simulink model "moore_machine"  (R2020a)
settings: Solver=VariableStepAuto  StartTime=0.0  StopTime=20  RelTol=1e-3
settings Model: Creator=macharold  LastModifiedBy=Roland Varga
settings DataIOCC: FinalStateName=myOperPoint  InitialState=myOperPoint  LoadExternalInput=on  SaveFinalState=on  SaveOperatingPoint=on  ReturnWorkspaceOutputs=off
settings DebuggingCC: SignalResolutionControl=None  ArithmeticOperatorsInVariantConditions=warning
settings SFSimCC: SimUseLocalCustomCode=off  CustomCodeUndefinedFunction=UseInterfaceOnly
settings RTWCC: RTWUseLocalCustomCode=off

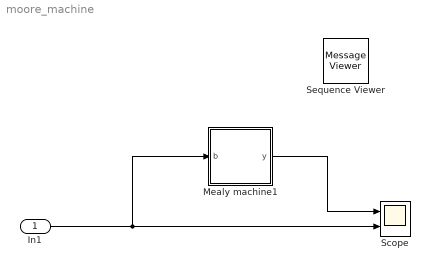
== system moore_machine ==
  In1 : Inport  SampleTime=1
  Mealy machine1 : Stateflow chart  TreatAsAtomicUnit=on
  Scope : Scope  NumInputPorts=2
  Sequence Viewer : MessageViewer  History=1000
  wires:
  In1/1 -> Mealy machine1/1(b), Scope/2
  Mealy machine1/1(y) -> Scope/1

== stateflow chart moore_machine/Mealy machine1 ==
  settings: sampleTime=1
  state S21
  state S20
  state S19
  state S1
  state S5
  state S6
  state S7
  state S8
  state S9
  state S10
  state S24
  state S25
  state S22
  state S14
  state S11
  state S13
  state S12
  state S26
  state S23
  state S15
  state S18
  state S17
  state S16
  state S28
  state S30
  state S31
  state S33
  state S34
  state S35
  state S36
  state S37
  state S38
  S16 -> S8 [order 1] : [b==1]{y=0}
  S21 -> S28 [order 2] : [b==0]{y=0}
  S19 -> S21 [order 2] : [b==1]
  S21 -> S13 [order 1] : [b==1]{y=0}
  S20 -> S28 [order 2] : [b==0]{y=0}
  S10 -> S19 [order 2] : [b==0]
  S19 -> S20 [order 1] : [b==0]
  S20 -> S18 [order 1] : [b==1]{y=0}
  S10 -> S10 [order 1] : [b==1]
  S1 -> S5 [order 2] : [b==1]
  S5 -> S6 [order 1] : [b==1]
  S6 -> S7 [order 1] : [b==1]{y=0}
  S7 -> S8 [order 1] : [b==1]
  S8 -> S9 [order 1] : [b==1]
  (default) -> S1 : {y=-1}
  S9 -> S10 [order 1] : [b==1]{y=1}
  S9 -> S14 [order 2] : [b==0]
  S31 -> S7 [order 2] : [b==1]
  S5 -> S26 [order 2] : [b==0]
  S1 -> S24 [order 1] : [b==0]
  S6 -> S28 [order 2] : [b==0]{y=0}
  S8 -> S14 [order 2] : [b==0]
  S7 -> S14 [order 2] : [b==0]
  S22 -> S9 [order 1] : [b==1]{y=0}
  S22 -> S14 [order 2] : [b==0]{y=0}
  S38 -> S24 [order 1] : [b==0]{y=-1}
  S24 -> S25 [order 2] : [b==1]
  S12 -> S22 [order 1] : [b==1]
  S24 -> S24 [order 1] : [b==0]
  S25 -> S31 [order 1] : [b==1]{y=0}
  S26 -> S24 [order 1] : [b==0]
  S25 -> S26 [order 2] : [b==0]
  S13 -> S12 [order 1] : [b==1]{y=1}
  S14 -> S11 [order 1] : [b==1]
  S16 -> S14 [order 2] : [b==0]{y=0}
  S11 -> S13 [order 1] : [b==1]
  S13 -> S28 [order 2] : [b==0]
  S11 -> S30 [order 2] : [b==0]
  S14 -> S15 [order 2] : [b==0]
  S23 -> S11 [order 2] : [b==1]{y=0}
  S12 -> S23 [order 2] : [b==0]
  S26 -> S30 [order 2] : [b==1]{y=0}
  S23 -> S15 [order 1] : [b==0]{y=0}
  S15 -> S28 [order 2] : [b==0]
  S15 -> S18 [order 1] : [b==1]
  S18 -> S17 [order 1] : [b==1]
  S17 -> S16 [order 1] : [b==1]{y=1}
  S17 -> S28 [order 2] : [b==0]
  S18 -> S30 [order 2] : [b==0]
  S28 -> S30 [order 1] : [b==1]
  S30 -> S31 [order 1] : [b==1]
  S28 -> S33 [order 2] : [b==0]
  S38 -> S30 [order 2] : [b==1]
  S37 -> S30 [order 2] : [b==1]
  S36 -> S30 [order 2] : [b==1]
  S34 -> S30 [order 2] : [b==1]
  S33 -> S30 [order 2] : [b==1]
  S35 -> S30 [order 2] : [b==1]
  S30 -> S33 [order 2] : [b==0]
  S31 -> S33 [order 1] : [b==0]
  S33 -> S34 [order 1] : [b==0]
  S34 -> S35 [order 1] : [b==0]
  S35 -> S36 [order 1] : [b==0]
  S36 -> S37 [order 1] : [b==0]
  S37 -> S38 [order 1] : [b==0]
  data: b input; y output
